simulink model "FLCU_Gauging_Test_Harness_Mass"  (R2019b)
settings: Solver=FixedStepAuto  StartTime=0.0  StopTime=10  FixedStep=0.02  RelTol=1e-3
settings Model: DataDictionary=FLCU_Gauging.sldd  Creator=aymanouchker  LastModifiedBy=aymanouchker
settings DataIOCC: SignalLoggingName=BusData
settings OptimizationCC: DefaultParameterBehavior=Inlined  UseDivisionForNetSlopeComputation=on  GainParamInheritBuiltInType=on  UseFloatMulNetSlope=on  DefaultUnderspecifiedDataType=single  UseSpecifiedMinMax=on  InlineInvariantSignals=on  EnhancedBackFolding=on  CachingGlobalReferences=on  PassReuseOutputArgsAs=Individual arguments  StateBitsets=on  DataBitsets=on  ZeroExternalMemoryAtStartup=off  ZeroInternalMemoryAtStartup=off  NoFixptDivByZeroProtection=on  EfficientFloat2IntCast=on  LifeSpan=inf  OptimizeBlockOrder=speed  DifferentSizesBufferReuse=on  EfficientTunableParamExpr=on
settings DebuggingCC: SignalInfNanChecking=warning  IntegerOverflowMsg=error  ParameterTunabilityLossMsg=error  UniqueDataStoreMsg=error  AssertControl=DisableAll  StrictBusMsg=ErrorOnBusTreatedAsVector  SFUndirectedBroadcastEventsDiag=error
settings HardwareCC: ProdBitPerInt=16  ProdBitPerPointer=16  ProdBitPerSizeT=16  ProdBitPerPtrDiffT=16  ProdLargestAtomicFloat=None  ProdWordSize=16  ProdLongLongMode=on  ProdHWDeviceType=STMicroelectronics->ST10/Super10
settings SFSimCC: CompileTimeRecursionLimit=0  EnableRuntimeRecursion=off  MATLABDynamicMemAlloc=off
settings RTWCC: SystemTargetFile=ert.tlc  TemplateMakefile=ert_default_tmf  GenerateReport=on  BuildConfiguration=Faster Runs  IncludeHyperlinkInReport=on  LaunchReport=on  GenerateTraceInfo=on  GenerateTraceReport=on  GenerateTraceReportSl=on  GenerateTraceReportSf=on  GenerateTraceReportEml=on
settings CodeAppCC: ForceParamTrailComments=on  IgnoreCustomStorageClasses=off  IgnoreTestpoints=on  OperatorAnnotations=on  SimulinkDataObjDesc=on  SFDataObjDesc=on  MATLABFcnDesc=on  InsertBlockDesc=on  StateflowObjectComments=on  MATLABSourceComments=on  EnableCustomComments=on  ReqsInCode=on
settings ERTTargetCC: TargetLangStandard=C99 (ISO)  UtilityFuncGeneration=Shared location  GenerateSampleERTMain=on  CombineSignalStateStructs=on  SuppressErrorStatus=on  SupportAbsoluteTime=off  MultiInstanceERTCode=on  CodeInterfacePackaging=Reusable function  SupportNonFinite=off  ParenthesesLevel=Maximum  CastingMode=Standards  GenerateSharedConstants=off  InlinedParameterPlacement=NonHierarchical  ERTCustomFileTemplate=example_file_process.tlc  PreserveExpressionOrder=on  PreserveIfCondition=on  EnableSignedLeftShifts=off  EnableSignedRightShifts=off

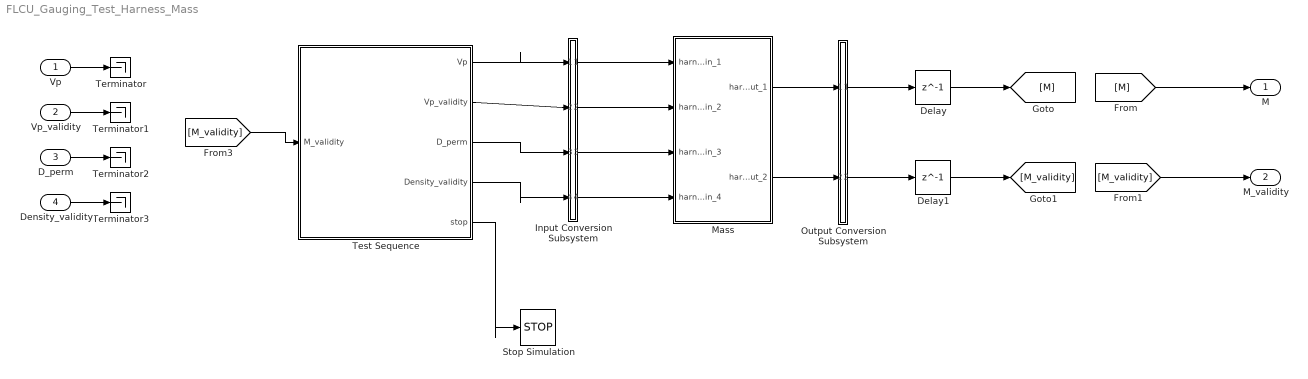
== system FLCU_Gauging_Test_Harness_Mass ==
  Vp : Inport  OutDataTypeStr=double  PortDimensions=[1]  SampleTime=0.02
  Vp_validity : Inport  Port=2  OutDataTypeStr=boolean  PortDimensions=[1]  SampleTime=0.02
  D_perm : Inport  Port=3  OutDataTypeStr=double  PortDimensions=[1]  SampleTime=[-1, 0]
  Density_validity : Inport  Port=4  OutDataTypeStr=boolean  PortDimensions=[1]  SampleTime=[-1, 0]
  Delay : Delay  DelayLength=1
  Delay1 : Delay  DelayLength=1
  Input Conversion Subsystem : Subsystem  Tag=__SLT_ICS__  Description=|
      | Signal spec.
      | and routing
      settings: AttributesFormatString=%<Description>
  Mass : Subsystem  Tag=__SL_testing_harness_stub_
  Output Conversion Subsystem : Subsystem  Tag=__SLT_OCS__  Description=|
      | Signal spec.
      | and routing
      settings: AttributesFormatString=%<Description>
  Stop Simulation : Stop
  Terminator{,1..3} (4 alike) : Terminator
  Test Sequence : Test Sequence  TreatAsAtomicUnit=on
  M : Outport
  M_validity : Outport  Port=2
  wires:
  Input Conversion Subsystem/1(Outport_1) -> Mass/1(harness_in_1)
  Input Conversion Subsystem/2(Outport_2) -> Mass/2(harness_in_2)
  Input Conversion Subsystem/3(Outport_3) -> Mass/3(harness_in_3)
  Input Conversion Subsystem/4(Outport_4) -> Mass/4(harness_in_4)
  Mass/1(harness_out_1) -> Output Conversion Subsystem/1(Inport_1)
  Mass/2(harness_out_2) -> Output Conversion Subsystem/2(Inport_2)
  Vp/1 -> Terminator/1
  Vp_validity/1 -> Terminator1/1
  D_perm/1 -> Terminator2/1
  Density_validity/1 -> Terminator3/1
  Output Conversion Subsystem/1(Outport_1) -> Delay/1
  Output Conversion Subsystem/2(Outport_2) -> Delay1/1
  Delay/1 -> [M]
  Delay1/1 -> [M_validity]
  [M_validity] -> M_validity/1
  [M] -> M/1
  [M_validity] -> Test Sequence/1(M_validity)
  Test Sequence/5(stop) -> Stop Simulation/1
  Test Sequence/4(Density_validity) -> Input Conversion Subsystem/4(Inport_4)
  Test Sequence/3(D_perm) -> Input Conversion Subsystem/3(Inport_3)
  Test Sequence/2(Vp_validity) -> Input Conversion Subsystem/2(Inport_2)
  Test Sequence/1(Vp) -> Input Conversion Subsystem/1(Inport_1)

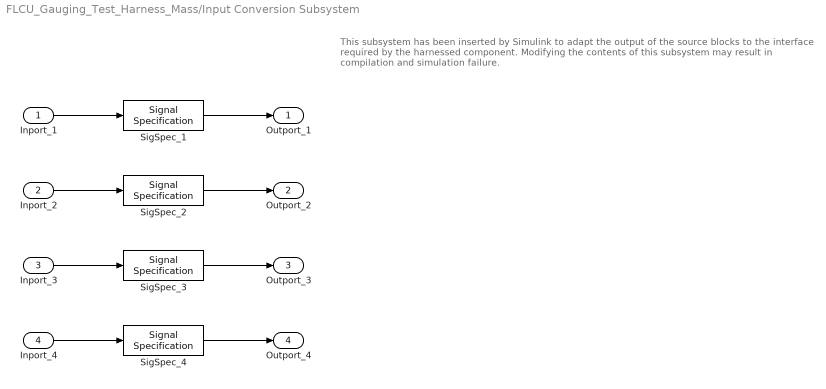
== system FLCU_Gauging_Test_Harness_Mass/Input Conversion Subsystem ==
  note: This subsystem has been inserted by Simulink to adapt the output of the source blocks to the interface required by the harnessed component.
      |  Modifying the contents of this subsystem may result in compilation and simulation failure.
  Inport_1 : Inport
  Inport_2 : Inport  Port=2
  Inport_3 : Inport  Port=3
  Inport_4 : Inport  Port=4
  SigSpec_1 : SignalSpecification  OutDataTypeStr=double  Unit=L  Dimensions=[1]  SampleTime=0.02
  SigSpec_2 : SignalSpecification  OutDataTypeStr=boolean  Dimensions=[1]  SampleTime=0.02
  SigSpec_3 : SignalSpecification  OutDataTypeStr=double  Unit=kg/L  Dimensions=[1]  SampleTime=[-1, 0]
  SigSpec_4 : SignalSpecification  OutDataTypeStr=boolean  Dimensions=[1]  SampleTime=[-1, 0]
  Outport_1 : Outport
  Outport_2 : Outport  Port=2
  Outport_3 : Outport  Port=3
  Outport_4 : Outport  Port=4
  wires:
  SigSpec_1/1 -> Outport_1/1
  Inport_1/1 -> SigSpec_1/1
  SigSpec_2/1 -> Outport_2/1
  Inport_2/1 -> SigSpec_2/1
  SigSpec_3/1 -> Outport_3/1
  Inport_3/1 -> SigSpec_3/1
  SigSpec_4/1 -> Outport_4/1
  Inport_4/1 -> SigSpec_4/1

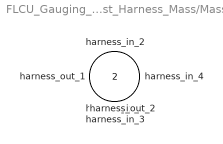
== system FLCU_Gauging_Test_Harness_Mass/Mass ==
  harness_in_1 : Inport
  harness_in_2 : Inport  Port=2
  harness_in_3 : Inport  Port=3
  harness_in_4 : Inport  Port=4
  harness_out_1 : Outport
  harness_out_2 : Outport  Port=2

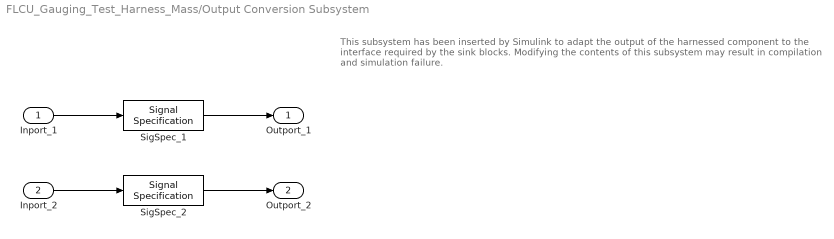
== system FLCU_Gauging_Test_Harness_Mass/Output Conversion Subsystem ==
  note: This subsystem has been inserted by Simulink to adapt the output of the harnessed component to the interface required by the sink blocks.
      |  Modifying the contents of this subsystem may result in compilation and simulation failure.
  Inport_1 : Inport
  Inport_2 : Inport  Port=2
  SigSpec_1 : SignalSpecification  OutDataTypeStr=double  Unit=kg  Dimensions=[1]  SampleTime=0.02
  SigSpec_2 : SignalSpecification  OutDataTypeStr=boolean  Dimensions=[1]  SampleTime=0.02
  Outport_1 : Outport
  Outport_2 : Outport  Port=2
  wires:
  Inport_1/1 -> SigSpec_1/1
  SigSpec_1/1 -> Outport_1/1
  Inport_2/1 -> SigSpec_2/1
  SigSpec_2/1 -> Outport_2/1

== stateflow chart FLCU_Gauging_Test_Harness_Mass/Test Sequence ==
  settings: stateMachineType=SIMPLIFIED_MACHINE
  state Initialization
    Vp=0;
    Vp_validity=true;
    D_perm=0;
    Density_validity=true;
    stop=false;
    count=0;
  state step_1
    Vp=110
    D_perm=0.80;
    Density_validity=true;
    Vp_validity=true;
  state step_2
    verify(M_validity==true);
  state step_3
    Vp=1;
    D_perm=1;
    Density_validity=true;
    Vp_validity=false;
  state step_4
    count=count+1;
    verify(M_validity==false);
  state step_5
    Vp=140;
    Vp_validity=false;
    D_perm=0.8;
    Density_validity=true;
  state step_6
    Vp=1;
    Vp_validity=true;
    D_perm=1;
    Density_validity=false;
  state step_7
    Vp=1;
    Vp_validity=false;
    D_perm=1;
    Density_validity=false;
  state step_8
    Vp=-100000;
    Vp_validity=true;
    D_perm=1;
    Density_validity=true;
  state step_9
    Vp=1;
    Vp_validity=true;
    D_perm=-100000;
    Density_validity=true;
  state step_10
    stop=true;
  (default) -> Initialization
  Initialization -> step_1
  step_1 -> step_2
  step_2 -> step_3
  step_3 -> step_4
  (junction 91) -> step_4
  (junction 116) -> (junction 91)
  step_4 -> (junction 145) [order 2] : [
      | count==2
      | ]
  (junction 145) -> (junction 128)
  step_4 -> (junction 148) [order 3] : [
      | count==3
      | ]
  (junction 148) -> (junction 132)
  step_4 -> (junction 153) [order 4] : [
      | count==4
      | ]
  (junction 153) -> (junction 136)
  step_4 -> (junction 168) [order 5] : [
      | count==5
      | ]
  (junction 168) -> (junction 166)
  step_4 -> (junction 173) [order 6] : [
      | count==6
      | ]
  (junction 173) -> (junction 171)
  step_4 -> step_5 [order 1] : [
      | count==1
      | ]
  step_5 -> step_4
  (junction 128) -> step_6
  step_6 -> (junction 116)
  (junction 118) -> (junction 116)
  (junction 132) -> step_7
  step_7 -> (junction 118)
  (junction 120) -> (junction 118)
  (junction 136) -> step_8
  step_8 -> (junction 120)
  (junction 166) -> step_9
  (junction 171) -> step_10
  data: M_validity input; count local; Vp output; Vp_validity output; D_perm output; Density_validity output; stop output
